simulink library "AR_Drone_Video_Processing"  (R2016a)
settings: Solver=ode45  StartTime=0.0  StopTime=10.0  RelTol=1e-3
settings Model: Creator=sannem  LastModifiedBy=sannem
settings DataIOCC: LimitDataPoints=on
settings DebuggingCC: AllowSymbolicDim=off

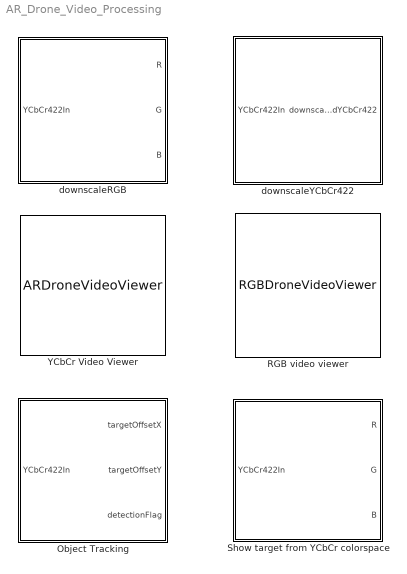
== system AR_Drone_Video_Processing ==
  Object Tracking : MATLAB Function  TreatAsAtomicUnit=on  mask(AR Drone:  Find Colored Object Position){width=1280, height=720, downScaleFactor=5, cbFloor=0, cbCeiling=117, crFloor=0, crCeiling=117, pixelThreshold=10}
      mask prompts: width "Video input width"; height "Video input height"; downScaleFactor "Video down sample factor"; cbFloor "Blue shift minimum [0-255]"; cbCeiling "Blue shift maximum [0-255]"; crFloor "Red shift minimum [0-255]"; crCeiling "Red shift maximum [0-255]"; pixelThreshold "Minimum object detection pixel count"
      mask help:
      | This MATLAB function block takes an input video stream, down samples in both the horizontal and veritcal direction to reduce the computational demand, and then determines how many pixels fall within the user specified colorspace region and what their average postition is in the video. If you are experiencing some artifacts which are hard to tune out, increase the minimum target pixel count. No target will be registered (detectionFlag = 0) unless as many pixels as you define are found in the target colorspace (detectionFlag = 1).
      | The output x and y position are scaled between -1 and 1.
      |
      | Using the YCbCr colorspace some recommend values are:
      |
      | Green target:
      | cb[min, max] = [0, 100]
      | cr[min, max] = [0, 100]
      |
      | Blue target:
      | cb[min, max] = [155, 255]
      | cr[min, max] = [0, 100]
      |
      | Red target:
      | cb[min, max] = [0, 100]
      | cr[min, max] = [155, 255]
  RGB video viewer : M-S-Function  FunctionName=RGBDroneVideoViewer  mask(ARDrone: RGB Video viewer){}
      mask help: This block will display video from incoming matrixes of unsigned 8 bit integers for the red, green and blue values of the video stream. This block works as an interface between the AR Drone and Simulink showing the video stream and therefor only works in external mode.
      mask Display:
      | disp('RGB Video viewer\n\n\n')
      | port_label('input',1,'R')
      | port_label('input',2,'G')
      | port_label('input',3,'B')
  Show target from YCbCr colorspace : MATLAB Function  TreatAsAtomicUnit=on  mask(ARDrone: Find Target In YCbCr Colorspace){width=1280, height=720, downScaleFactor=5, cbFloor=0, cbCeiling=118, crFloor=0, crCeiling=118, pixelThreshold=10}
      mask prompts: width "Video input width"; height "Video input height"; downScaleFactor "Video downsample factor"; cbFloor "Blue shift minimum [0-255]"; cbCeiling "Blue shift maximum [0-255]"; crFloor "Red shift minimum [0-255]"; crCeiling "Red shift maximum [0-255]"; pixelThreshold "Minimum object detection pixel count"
      mask help:
      | This MATLAB function block takes an input video stream, down samples in both the horizontal and veritcal direction to reduce the computational demand, and then determines how many pixels fall within the user specified colorspace region and what their average postition is in the video. If you are experiencing some artifacts which are hard to tune out, increase the minimum target pixel count. No target will be registered unless as many pixels as you define are found in the target colorspace.
      |
      | Using the YCbCr colorspace some recommend values are:
      |
      | Green target:
      | cb[min, max] = [0, 100]
      | cr[min, max] = [0, 100]
      |
      | Blue target:
      | cb[min, max] = [155, 255]
      | cr[min, max] = [0, 100]
      |
      | Red target:
      | cb[min, max] = [0, 100]
      | cr[min, max] = [155, 255]
  YCbCr Video Viewer : M-S-Function  FunctionName=ARDroneVideoViewer  Parameters=horAspect,verAspect  mask(YCbCr Video viewer){horAspect=16, verAspect=9}
      mask prompts: horAspect "Horizontal video aspect ratio"; verAspect "Vertical video aspect ratio"
      mask help: This block allows YCbCr colorspace, 4:2:2 subpixels video sources, such as the AR Drone 2.0 camera's to be shown. This block works as an interface between the AR Drone and Simulink showing the video stream and therefor only works in external mode.
      mask Display:
      | disp('YCbCr Video viewer\n\n\n')
      | port_label('input',1,'Video in');
  "downscaleRGB " : MATLAB Function  TreatAsAtomicUnit=on  mask(ARDrone: Down scale to RGB){width=1280, height=720, downScaleFactor=8}
      mask prompts: width "Input Image width"; height "Input Image height"; downScaleFactor "Down scaling factor"
      mask help: This Block downscales and converts an YCrCb input stream to RGB and outputs it as matrixes of intensity values.
  downscaleYCbCr422 : MATLAB Function  TreatAsAtomicUnit=on  mask(Down scaled chromatic){width=1280, height=720, downScaleFactor=8}
      mask prompts: width "Input Image width"; height "Input Image height"; downScaleFactor "Down scaling factor"
      mask help: This Block downscales the chromatic value of a YCrCb input stream and outputs it as a matrix of intensity values

== matlab function AR_Drone_Video_Processing/downscaleRGB  ==
  data: YCbCr422In input; R output; width parameter; height parameter; downScaleFactor parameter; G output; B output

function [R,G,B]   = downscaleRGB(YCbCr422In,width, height, downScaleFactor)
 
R = uint8(zeros(height/downScaleFactor,width/downScaleFactor));
G = uint8(zeros(height/downScaleFactor,width/downScaleFactor));
B = uint8(zeros(height/downScaleFactor,width/downScaleFactor));
if ~isempty(YCbCr422In)

    %% constants for color conversion
    c1 =     298.082/256;
    Rc1 =    408.583/256;
    Rc2 =   -222.921;
    Gc1 =   -100.291/256;
    Gc2 =   -208.120/256;
    Gc3 =    135.576;
    Bc1=     516.412/256;
    Bc2=    -276.836;

    %% Downsample and convert to RGB

    for verticalIndex = 1 : 1 : height/downScaleFactor;             % indexing for downsampled vertical direction
        for horizontalIndex = 1 : 1 : (width / 2)/downScaleFactor;  % indexing for downsampled horizontal direction
            index = 4 * (downScaleFactor * (verticalIndex - 1) * (width / 2) + downScaleFactor * horizontalIndex) - 3;  % translate the horizontal and vertical indexes into the index into the video input
            pixel = [single(YCbCr422In(index)) single(YCbCr422In(index+1)) single(YCbCr422In(index+2)) single(YCbCr422In(index+3))];
            R(verticalIndex, 2 * horizontalIndex - 1) = c1 * pixel(2) + Rc1 * pixel(3) + Rc2;
            G(verticalIndex, 2 * horizontalIndex - 1) = c1 * pixel(2) + Gc1 * pixel(1) + Gc2 * pixel(3) + Gc3;
            B(verticalIndex, 2 * horizontalIndex - 1) = c1 * pixel(2) + Bc1 * pixel(1) + Bc2;
            R(verticalIndex, 2 * horizontalIndex) = c1 * pixel(4) + Rc1 * pixel(3) + Rc2;
            G(verticalIndex, 2 * horizontalIndex) = c1 * pixel(4) + Gc1 * pixel(1) + Gc2 * pixel(3) + Gc3;
            B(verticalIndex, 2 * horizontalIndex) = c1 * pixel(4) + Bc1 * pixel(1) + Bc2;
        end
    end
end
end

== matlab function AR_Drone_Video_Processing/downscaleYCbCr422 ==
  data: YCbCr422In input; downscaledYCbCr422 output; width parameter; height parameter; downScaleFactor parameter

function downscaledYCbCr422    = downscaleYCbCr422(YCbCr422In, width, height, downScaleFactor)

%% Downsample and convert to RGB

outputLength = width * height * 2 / downScaleFactor / downScaleFactor;
downscaledYCbCr422 = uint8( zeros( outputLength, 1) );

outputIndex = 1;
for verticalIndex = 1 : 1 : height/downScaleFactor;             % indexing for downsampled vertical direction
    for horizontalIndex = 1 : 1 : (width / 2)/downScaleFactor;  % indexing for downsampled horizontal direction
        index = 4 * (downScaleFactor * (verticalIndex - 1) * (width / 2) + downScaleFactor * horizontalIndex) - 3;  % translate the horizontal and vertical indexes into the index into the video input
        downscaledYCbCr422(outputIndex : outputIndex + 3) = uint8(YCbCr422In(index : index + 3));
        outputIndex = outputIndex + 4;
    end
end
end

== matlab function AR_Drone_Video_Processing/Object Tracking ==
  data: YCbCr422In input; targetOffsetX output; targetOffsetY output; detectionFlag output; cbFloor parameter; cbCeiling parameter; crFloor parameter; crCeiling parameter; downScaleFactor parameter; height parameter; width parameter; pixelThreshold parameter
function [targetOffsetX, targetOffsetY, detectionFlag]  = coloredObjectPosition(YCbCr422In,cbFloor, cbCeiling, crFloor, crCeiling, downScaleFactor, height, width, pixelThreshold)

xPositionSum = 0;
yPositionSum = 0;
targetOffsetX = 0;
targetOffsetY = 0;
targetPixelCount = 0;
detectionFlag = 0;

for verticalIndex = 1 : 1 : height/downScaleFactor;             % indexing for downsampled vertical direction
    for horizontalIndex = 1 : 1 : (width / 2)/downScaleFactor;  % indexing for downsampled horizontal direction
        index = 4 * (downScaleFactor * (verticalIndex - 1) * (width / 2) + downScaleFactor * horizontalIndex) - 3;  % translate the horizontal and vertical indexes into the index into the video input
        pixel = double([YCbCr422In(index) YCbCr422In(index+1) YCbCr422In(index+2) YCbCr422In(index+3)]);    % retrieve the pixel data and convert for calculation

        %% verify whether this pixel is within the user specified region of the YCbCr colorspace
        if ( pixel(1)  >= cbFloor && pixel(1)  <= cbCeiling && ...
             pixel(3)  >= crFloor && pixel(3)  <= crCeiling  )

            targetPixelCount = targetPixelCount + 1;
            xPositionSum = xPositionSum + 2 * horizontalIndex * downScaleFactor;
            yPositionSum = yPositionSum + verticalIndex * downScaleFactor;
        end
    end
end

% compute the average green pixel position
if targetPixelCount > pixelThreshold
    detectionFlag = 1;
    targetOffsetX = xPositionSum / targetPixelCount / (0.5 * width) - 1;     
    targetOffsetY = -(yPositionSum / targetPixelCount / (0.5 * height) - 1);
else
    % not enough pixels were target pixels:

end

end

== matlab function AR_Drone_Video_Processing/Show target from YCbCr colorspace ==
  data: YCbCr422In input; cbFloor parameter; cbCeiling parameter; crFloor parameter; crCeiling parameter; downScaleFactor parameter; height parameter; width parameter; R output; G output; B output; pixelThreshold parameter
function [R, G, B]  = showYCbCrTarget(YCbCr422In,cbFloor, cbCeiling, crFloor, crCeiling, downScaleFactor, height, width, pixelThreshold)

xPositionSum = 0;
yPositionSum = 0;
xPositionMean = -1;
yPositionMean = -1;
targetPixelCount = 0;

%% create a 'RGB' matrix for showing the detected pixels
R = uint8(zeros((width / 2)/downScaleFactor, height/downScaleFactor));

for verticalIndex = 1 : 1 : height/downScaleFactor;             % indexing for downsampled vertical direction
    for horizontalIndex = 1 : 1 : (width / 2)/downScaleFactor;  % indexing for downsampled horizontal direction
        index = 4 * (downScaleFactor * (verticalIndex - 1) * (width / 2) + downScaleFactor * horizontalIndex) - 3;  % translate the horizontal and vertical indexes into the index into the video input
        pixel = double([YCbCr422In(index) YCbCr422In(index+1) YCbCr422In(index+2) YCbCr422In(index+3)]);    % retrieve the pixel data and convert for calculation

        %% verify whether this pixel is within the user specified region of the YCbCr colorspace
        if ( pixel(1)  >= cbFloor && pixel(1)  <= cbCeiling && ...
             pixel(3)  >= crFloor && pixel(3)  <= crCeiling  )

            targetPixelCount = targetPixelCount + 1;
            xPositionSum = xPositionSum + horizontalIndex * downScaleFactor;
            yPositionSum = yPositionSum + verticalIndex * downScaleFactor;
            % set the targetView
            R(horizontalIndex,verticalIndex) = uint8(255);

        end
    end
end

% compute the average green pixel position
if targetPixelCount > pixelThreshold
    % copy the target view to B and G such it becomes white
    B = R;
    G = R;
    xPositionMean = xPositionSum / targetPixelCount;     
    yPositionMean = yPositionSum / targetPixelCount;
    % mark this position as a red pixel
    xScale = xPositionMean / downScaleFactor;
    yScale = yPositionMean / downScaleFactor;
    R(floor(xScale),floor(yScale)) = uint8(255);
    G(floor(xScale),floor(yScale)) = 0;
    B(floor(xScale),floor(yScale)) = 0;
else
    % not enough pixels were target pixels so reset R
    R = uint8(zeros((width / 2)/downScaleFactor, height/downScaleFactor));
    B = R;
    G = R;
end

end
